simulink model "exercise_02_simscape"  (R2022b)
settings: Solver=VariableStepAuto  StartTime=0.0  StopTime=10*2*pi/w  MaxStep=1e-4  MinStep=1e-12  RelTol=1e-3  AbsTol=1e-3
model workspace (MAT data in the model file):
  R = 0.5
  X1 = 1
  X2 = 2
  XC = -1
  XM = 1
  phase_curr1 = -0.785398163397
  phase_curr2 = 3.14159265359
  value_curr1 = 1.41421356237
  value_curr2 = 4
  w = 6.28318530718
libraries: fl_lib x19, nesl_utility x4
settings Model: Creator=paolo  LastModifiedBy=stefa
settings SolverCC: AutoScaleAbsTol=off  AlgebraicLoopSolver=TrustRegion  MaxZcPerStep=1
settings DebuggingCC: UnconnectedInputMsg=warning  UnconnectedOutputMsg=warning  UnconnectedLineMsg=warning  SymbolicDimsDataTypeCodeGenerationDiagnostic=none
settings ModelReferenceCC: EnableRefExpFcnMdlSchedulingChecks=on
settings SFSimCC: CustomCodeUndefinedFunction=UseInterfaceOnly
settings RTWCC: DLArmComputeVersion=19.05
settings SimscapeCC: SimscapeLogType=all  SimscapeLogSimulationStatistics=on  SimscapeLogDataHistory=10000

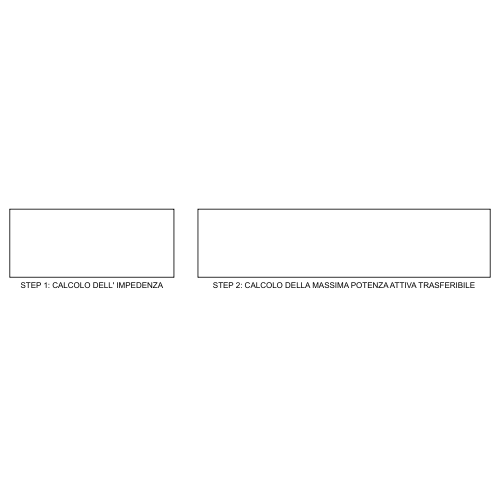
[thumbnail: Simulink's stored preview of the top-level diagram]
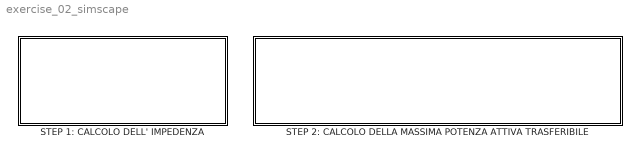
== system exercise_02_simscape ==
  STEP 1: CALCOLO DELL' IMPEDENZA : Subsystem
  STEP 2: CALCOLO DELLA MASSIMA POTENZA ATTIVA TRASFERIBILE : Subsystem

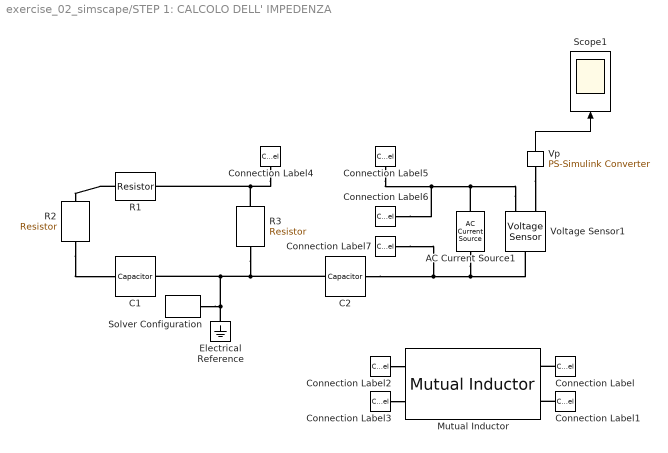
== system exercise_02_simscape/STEP 1: CALCOLO DELL' IMPEDENZA ==
  AC Current Source1 : fl_lib/Electrical/Electrical Sources/AC Current Source  amp=1 A  shift=pi/2 rad  frequency=w/(2*pi) Hz  omega=0 rad/s
      settings: InternalSimscapePortConfiguration="{\"Bottom\":[],\"Left\":[{\"id\":\"p\",\"label\":\"\",\"type\":\"foundation.electrical.electrical\"}],\"Right\":[{\"id\":\"n\",\"label\":\"\",\"type\":\"foundation.electrical.electrical\"}],\"Top\":[]}"
  C1 : fl_lib/Electrical/Electrical Elements/Capacitor  c=-1/w*XC F  r=0 Ohm  g=0 1/Ohm  i_specify=off  i_priority=None  i=0 A  i_nominal_specify=off  i_nominal_unit=A  i_nominal_value=1  v_specify=off  v_priority=None  v=0 V  v_nominal_specify=off  v_nominal_unit=V  v_nominal_value=1  vc_specify=off  vc_priority=High  vc=0 V  vc_nominal_specify=off  vc_nominal_unit=V  vc_nominal_value=1
  C2 : fl_lib/Electrical/Electrical Elements/Capacitor  c=-1/w*XC F  r=0 Ohm  g=0 1/Ohm  i_specify=off  i_priority=None  i=0 A  i_nominal_specify=off  i_nominal_unit=A  i_nominal_value=1  v_specify=off  v_priority=None  v=0 V  v_nominal_specify=off  v_nominal_unit=V  v_nominal_value=1  vc_specify=off  vc_priority=High  vc=0 V  vc_nominal_specify=off  vc_nominal_unit=V  vc_nominal_value=1
  Connection Label : ConnectionLabel  Label=induttore2_positivo
  Connection Label1 : ConnectionLabel  Label=induttore2_negativo
  Connection Label2 : ConnectionLabel  Label=induttore1_positivo
  Connection Label3 : ConnectionLabel  Label=induttore1_negativo
  Connection Label4 : ConnectionLabel  Label=induttore1_negativo
  Connection Label5 : ConnectionLabel  Label=induttore1_positivo
  Connection Label6 : ConnectionLabel  Label=induttore2_positivo
  Connection Label7 : ConnectionLabel  Label=induttore2_negativo
  Electrical Reference : fl_lib/Electrical/Electrical Elements/Electrical Reference
  Mutual Inductor : fl_lib/Electrical/Electrical Elements/Mutual Inductor  L1=X1/w H  L2=X2/w H  k=XM/sqrt(X1*X2)  i1_specify=off  i1_priority=High  i1=0 A  i1_nominal_specify=off  i1_nominal_unit=A  i1_nominal_value=1  i2_specify=off  i2_priority=High  i2=0 A  i2_nominal_specify=off  i2_nominal_unit=A  i2_nominal_value=1  v1_specify=off  v1_priority=None  v1=0 V  v1_nominal_specify=off  v1_nominal_unit=V  v1_nominal_value=1  v2_specify=off  v2_priority=None  v2=0 V  v2_nominal_specify=off  v2_nominal_unit=V  v2_nominal_value=1
      settings: InternalSimscapePortConfiguration="{\"Bottom\":[],\"Left\":[{\"id\":\"p1\",\"label\":\"1+\",\"type\":\"foundation.electrical.electrical\"},{\"id\":\"n1\",\"label\":\"1-\",\"type\":\"foundation.electrical.electrical\"}],\"Right\":[{\"id\":\"p2\",\"label\":\"2+\",\"type\":\"foundation.electrical.electrical\"},{\"id\":\"n2\",\"label\":\"2-\",\"type\":\"foundation.electrical.electrical\"}],\"Top\":[]}"
  R1 : fl_lib/Electrical/Electrical Elements/Resistor  R=R Ohm  i_specify=off  i_priority=None  i=0 A  i_nominal_specify=off  i_nominal_unit=A  i_nominal_value=1  v_specify=off  v_priority=None  v=0 V  v_nominal_specify=off  v_nominal_unit=V  v_nominal_value=1
  R2 : fl_lib/Electrical/Electrical Elements/Resistor  R=R Ohm  i_specify=off  i_priority=None  i=0 A  i_nominal_specify=off  i_nominal_unit=A  i_nominal_value=1  v_specify=off  v_priority=None  v=0 V  v_nominal_specify=off  v_nominal_unit=V  v_nominal_value=1
  R3 : fl_lib/Electrical/Electrical Elements/Resistor  R=R Ohm  i_specify=off  i_priority=None  i=0 A  i_nominal_specify=off  i_nominal_unit=A  i_nominal_value=1  v_specify=off  v_priority=None  v=0 V  v_nominal_specify=off  v_nominal_unit=V  v_nominal_value=1
  Scope1 : Scope
  Solver Configuration : nesl_utility/Solver Configuration  PhysicalDomain=network_engine_domain  SubClassName=solver  LeftPortType=input  RightPortType=generic  Tones=[]  Harmonics=[]  SimulateNoise=off  Profile=off  UseLocalSampling=off  EnableSwitchedLinearOptims=on  FrequencyDomain=off  UseCCode=off  RelTol=0.001  AbsTol=0.001  MinStep=1e-09  ToWorkspace=off  RevertToSquareIcSolve=off  NumHomotopyIterations=100  PhasorMode=off  PhasorModeNumHarmonics=1  ConsistencySolver=NEWTON_XTOL_AFTER_FTOL  IndexReductionMethod=DerivativeReplacement  DoDC=off  ResidualTolerance=1e-09  ConsistencyTolSource=GLOBAL  ConsistencyAbsTol=0.001  ConsistencyRelTol=0.001  ConsistencyTolFactor=0.001  UseLocalSolver=off  LocalSolverChoice=NE_BACKWARD_EULER_ADVANCER  ResolveIndetEquations=on  FunctionEvalNumThread=1  LocalSolverSampleTime=0.001  DoFixedCost=off  MaxNonlinIter=3  MaxModeIter=2  ComputeImpulses=off  ImpulseIterations=2  LinearAlgebra=auto  LinearAlgebraNumThread=0  EquationFormulation=NE_TIME_EF  DelaysMemoryBudget=1024  AutomaticFiltering=on  FilteringTimeConstant=0.001  PartitionStorageMethod=AS_NEEDED  PartitionMemoryBudget=1024  PartitionMethod=ROBUST
  Voltage Sensor1 : fl_lib/Electrical/Electrical Sensors/Voltage Sensor
  Vp : nesl_utility/PS-Simulink Converter  PhysicalDomain=network_engine_domain  SubClassName=ps_output  LeftPortType=input  RightPortType=output  PseudoPeriodic=off  Frequencies=[]  VectorFormat=1-D array  Unit=inherit  AffineConversion=off
  wires:
  Vp/1 -> Scope1/1
  connections:
  Vp/LConn1 -- Voltage Sensor1/RConn1
  Voltage Sensor1/RConn2 -- AC Current Source1/RConn1 -- Connection Label6/LConn1 -- Connection Label5/LConn1
  AC Current Source1/LConn1 -- Connection Label7/LConn1 -- C2/RConn1 -- Voltage Sensor1/LConn1
  R1/RConn1 -- Connection Label4/LConn1 -- R3/LConn1
  R2/RConn1 -- C1/LConn1
  C1/RConn1 -- Electrical Reference/LConn1 -- Solver Configuration/RConn1 -- R3/RConn1 -- C2/LConn1
  Connection Label/LConn1 -- Mutual Inductor/RConn1
  Connection Label1/LConn1 -- Mutual Inductor/RConn2
  Connection Label2/LConn1 -- Mutual Inductor/LConn1
  Connection Label3/LConn1 -- Mutual Inductor/LConn2
  R1/LConn1 -- R2/LConn1

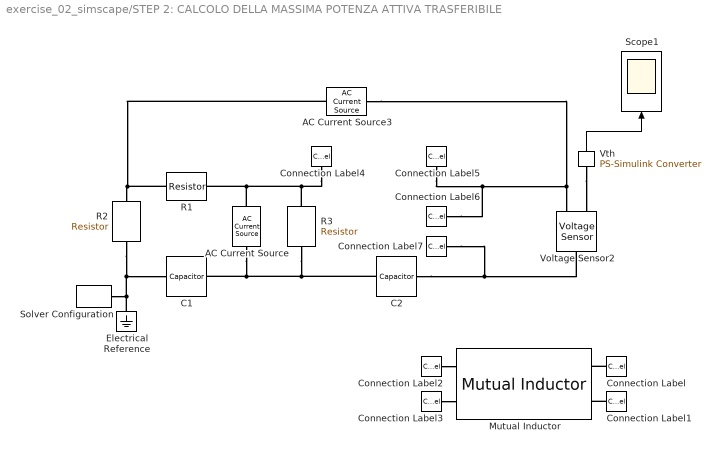
== system exercise_02_simscape/STEP 2: CALCOLO DELLA MASSIMA POTENZA ATTIVA TRASFERIBILE ==
  AC Current Source : fl_lib/Electrical/Electrical Sources/AC Current Source  amp=value_curr1*sqrt(2) A  shift=pi/2 + phase_curr1 rad  frequency=w/(2*pi) Hz  omega=0 rad/s
      settings: LibrarySourceBlock=simscape/STEP 1: CALCOLO DELL' IMPEDENZA/AC Current Source  InternalSimscapePortConfiguration="{\"Bottom\":[],\"Left\":[{\"id\":\"p\",\"label\":\"\",\"type\":\"foundation.electrical.electrical\"}],\"Right\":[{\"id\":\"n\",\"label\":\"\",\"type\":\"foundation.electrical.electrical\"}],\"Top\":[]}"
  AC Current Source3 : fl_lib/Electrical/Electrical Sources/AC Current Source  amp=value_curr2*sqrt(2) A  shift=pi/2 + phase_curr2 rad  frequency=w/(2*pi) Hz  omega=0 rad/s
      settings: LibrarySourceBlock=simscape/STEP 1: CALCOLO DELL' IMPEDENZA/AC Current Source2  InternalSimscapePortConfiguration="{\"Bottom\":[],\"Left\":[{\"id\":\"p\",\"label\":\"\",\"type\":\"foundation.electrical.electrical\"}],\"Right\":[{\"id\":\"n\",\"label\":\"\",\"type\":\"foundation.electrical.electrical\"}],\"Top\":[]}"
  C1 : fl_lib/Electrical/Electrical Elements/Capacitor  c=-1/w*XC F  r=0 Ohm  g=0 1/Ohm  i_specify=off  i_priority=None  i=0 A  i_nominal_specify=off  i_nominal_unit=A  i_nominal_value=1  v_specify=off  v_priority=None  v=0 V  v_nominal_specify=off  v_nominal_unit=V  v_nominal_value=1  vc_specify=off  vc_priority=High  vc=0 V  vc_nominal_specify=off  vc_nominal_unit=V  vc_nominal_value=1
      settings: LibrarySourceBlock=simscape/STEP 1: CALCOLO DELL' IMPEDENZA/C1
  C2 : fl_lib/Electrical/Electrical Elements/Capacitor  c=-1/w*XC F  r=0 Ohm  g=0 1/Ohm  i_specify=off  i_priority=None  i=0 A  i_nominal_specify=off  i_nominal_unit=A  i_nominal_value=1  v_specify=off  v_priority=None  v=0 V  v_nominal_specify=off  v_nominal_unit=V  v_nominal_value=1  vc_specify=off  vc_priority=High  vc=0 V  vc_nominal_specify=off  vc_nominal_unit=V  vc_nominal_value=1
      settings: LibrarySourceBlock=simscape/STEP 1: CALCOLO DELL' IMPEDENZA/C2
  Connection Label : ConnectionLabel  Label=induttore2_positivo
  Connection Label1 : ConnectionLabel  Label=induttore2_negativo
  Connection Label2 : ConnectionLabel  Label=induttore1_positivo
  Connection Label3 : ConnectionLabel  Label=induttore1_negativo
  Connection Label4 : ConnectionLabel  Label=induttore1_negativo
  Connection Label5 : ConnectionLabel  Label=induttore1_positivo
  Connection Label6 : ConnectionLabel  Label=induttore2_positivo
  Connection Label7 : ConnectionLabel  Label=induttore2_negativo
  Electrical Reference : fl_lib/Electrical/Electrical Elements/Electrical Reference
      settings: LibrarySourceBlock=simscape/STEP 1: CALCOLO DELL' IMPEDENZA/Electrical Reference
  Mutual Inductor : fl_lib/Electrical/Electrical Elements/Mutual Inductor  L1=X1/w H  L2=X2/w H  k=XM/sqrt(X1*X2)  i1_specify=off  i1_priority=High  i1=0 A  i1_nominal_specify=off  i1_nominal_unit=A  i1_nominal_value=1  i2_specify=off  i2_priority=High  i2=0 A  i2_nominal_specify=off  i2_nominal_unit=A  i2_nominal_value=1  v1_specify=off  v1_priority=None  v1=0 V  v1_nominal_specify=off  v1_nominal_unit=V  v1_nominal_value=1  v2_specify=off  v2_priority=None  v2=0 V  v2_nominal_specify=off  v2_nominal_unit=V  v2_nominal_value=1
      settings: LibrarySourceBlock=simscape/STEP 1: CALCOLO DELL' IMPEDENZA/Mutual Inductor  InternalSimscapePortConfiguration="{\"Bottom\":[],\"Left\":[{\"id\":\"p1\",\"label\":\"1+\",\"type\":\"foundation.electrical.electrical\"},{\"id\":\"n1\",\"label\":\"1-\",\"type\":\"foundation.electrical.electrical\"}],\"Right\":[{\"id\":\"p2\",\"label\":\"2+\",\"type\":\"foundation.electrical.electrical\"},{\"id\":\"n2\",\"label\":\"2-\",\"type\":\"foundation.electrical.electrical\"}],\"Top\":[]}"
  R1 : fl_lib/Electrical/Electrical Elements/Resistor  R=R Ohm  i_specify=off  i_priority=None  i=0 A  i_nominal_specify=off  i_nominal_unit=A  i_nominal_value=1  v_specify=off  v_priority=None  v=0 V  v_nominal_specify=off  v_nominal_unit=V  v_nominal_value=1
      settings: LibrarySourceBlock=simscape/STEP 1: CALCOLO DELL' IMPEDENZA/R1
  R2 : fl_lib/Electrical/Electrical Elements/Resistor  R=R Ohm  i_specify=off  i_priority=None  i=0 A  i_nominal_specify=off  i_nominal_unit=A  i_nominal_value=1  v_specify=off  v_priority=None  v=0 V  v_nominal_specify=off  v_nominal_unit=V  v_nominal_value=1
      settings: LibrarySourceBlock=simscape/STEP 1: CALCOLO DELL' IMPEDENZA/R2
  R3 : fl_lib/Electrical/Electrical Elements/Resistor  R=R Ohm  i_specify=off  i_priority=None  i=0 A  i_nominal_specify=off  i_nominal_unit=A  i_nominal_value=1  v_specify=off  v_priority=None  v=0 V  v_nominal_specify=off  v_nominal_unit=V  v_nominal_value=1
      settings: LibrarySourceBlock=simscape/STEP 1: CALCOLO DELL' IMPEDENZA/R3
  Scope1 : Scope
  Solver Configuration : nesl_utility/Solver Configuration  PhysicalDomain=network_engine_domain  SubClassName=solver  LeftPortType=input  RightPortType=generic  Tones=[]  Harmonics=[]  SimulateNoise=off  Profile=off  UseLocalSampling=off  EnableSwitchedLinearOptims=on  FrequencyDomain=off  UseCCode=off  RelTol=0.001  AbsTol=0.001  MinStep=1e-09  ToWorkspace=off  RevertToSquareIcSolve=off  NumHomotopyIterations=100  PhasorMode=off  PhasorModeNumHarmonics=1  ConsistencySolver=NEWTON_XTOL_AFTER_FTOL  IndexReductionMethod=DerivativeReplacement  DoDC=off  ResidualTolerance=1e-09  ConsistencyTolSource=GLOBAL  ConsistencyAbsTol=0.001  ConsistencyRelTol=0.001  ConsistencyTolFactor=0.001  UseLocalSolver=off  LocalSolverChoice=NE_BACKWARD_EULER_ADVANCER  ResolveIndetEquations=on  FunctionEvalNumThread=1  LocalSolverSampleTime=0.001  DoFixedCost=off  MaxNonlinIter=3  MaxModeIter=2  ComputeImpulses=off  ImpulseIterations=2  LinearAlgebra=auto  LinearAlgebraNumThread=0  EquationFormulation=NE_TIME_EF  DelaysMemoryBudget=1024  AutomaticFiltering=on  FilteringTimeConstant=0.001  PartitionStorageMethod=AS_NEEDED  PartitionMemoryBudget=1024  PartitionMethod=ROBUST
      settings: LibrarySourceBlock=|
      | simscape/STEP 1: CALCOLO DELL' IMPEDENZA/Solver
      | Configuration
  Voltage Sensor2 : fl_lib/Electrical/Electrical Sensors/Voltage Sensor
      settings: LibrarySourceBlock=simscape/STEP 1: CALCOLO DELL' IMPEDENZA/Voltage Sensor1
  Vth : nesl_utility/PS-Simulink Converter  PhysicalDomain=network_engine_domain  SubClassName=ps_output  LeftPortType=input  RightPortType=output  PseudoPeriodic=off  Frequencies=[]  VectorFormat=1-D array  Unit=inherit  AffineConversion=off
      settings: LibrarySourceBlock=simscape/STEP 1: CALCOLO DELL' IMPEDENZA/Vp
  wires:
  Vth/1 -> Scope1/1
  connections:
  Voltage Sensor2/LConn1 -- Connection Label7/LConn1 -- C2/RConn1
  AC Current Source/RConn1 -- R3/RConn1 -- C2/LConn1 -- C1/RConn1
  Connection Label5/LConn1 -- Connection Label6/LConn1 -- Voltage Sensor2/RConn2 -- AC Current Source3/LConn1
  AC Current Source/LConn1 -- Connection Label4/LConn1 -- R3/LConn1 -- R1/RConn1
  R1/LConn1 -- AC Current Source3/RConn1 -- R2/LConn1
  Connection Label1/LConn1 -- Mutual Inductor/RConn2
  Connection Label2/LConn1 -- Mutual Inductor/LConn1
  Connection Label3/LConn1 -- Mutual Inductor/LConn2
  R2/RConn1 -- C1/LConn1 -- Solver Configuration/RConn1 -- Electrical Reference/LConn1
  Vth/LConn1 -- Voltage Sensor2/RConn1
  Connection Label/LConn1 -- Mutual Inductor/RConn1
